simulink model "hw1b"  (R2022b)
settings: Solver=VariableStepAuto  StartTime=0.0  StopTime=200.0  FixedStep=0.1  MaxStep=0.1  MinStep=0.001  RelTol=1e-5  AbsTol=1e-8
undefined symbols (not defined in the file or in its folder): orbit, sat
settings Model: Creator=gagandeepthapar  LastModifiedBy=gagandeepthapar
settings SolverCC: InitialStep=0.1

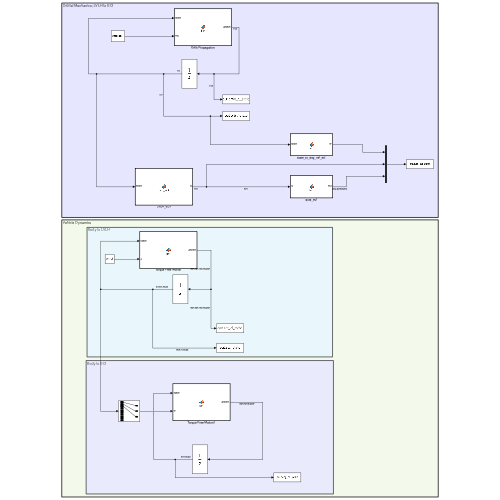
[thumbnail: Simulink's stored preview of the top-level diagram]
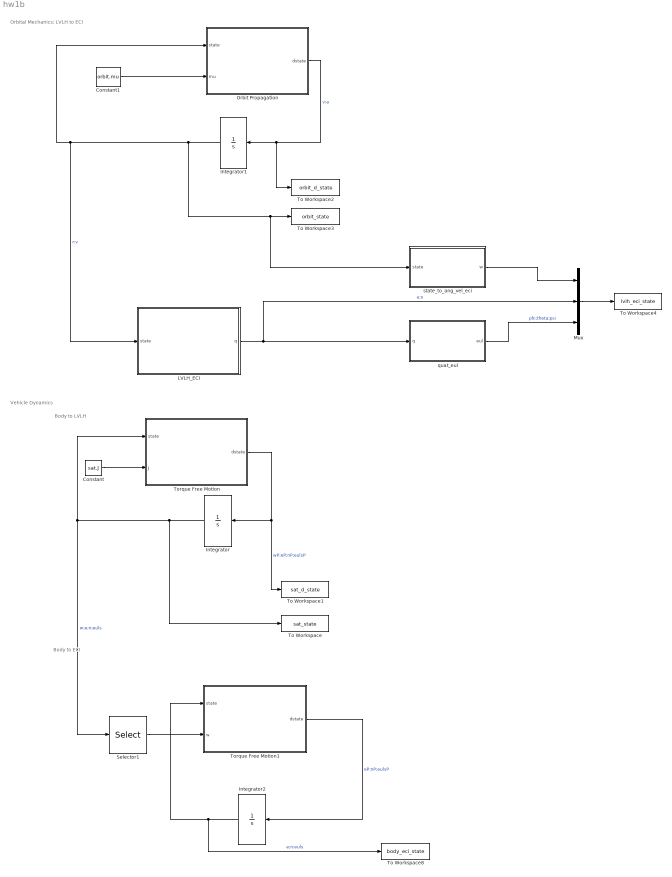
== system hw1b ==
  note: Body to LVLH
  note: Body to ECI
  note: Vehicle Dynamics
  note: Orbital Mechanics; LVLH to ECI
  Constant : Constant  Value=sat.J
  Constant1 : Constant  Value=orbit.mu
  Integrator : Integrator  InitialCondition=sat.state0
  Integrator1 : Integrator  InitialCondition=orbit.state0
  Integrator2 : Integrator  InitialCondition=sat.eci_state0
  LVLH_ECI : MATLAB Function  TreatAsAtomicUnit=on
  Mux : Mux  Inputs=3
  Orbit Propagation : MATLAB Function  TreatAsAtomicUnit=on
  Selector1 : Selector  InputPortWidth=10  IndexOptions=Index vector (dialog)  Indices=[1:3]  OutputSizes=1
  To Workspace : ToWorkspace  VariableName=sat_state  SampleTime=-1
      settings: Save2DSignal=2-D array (concatenate along first dimension)
  To Workspace1 : ToWorkspace  VariableName=sat_d_state  SampleTime=-1
      settings: Save2DSignal=2-D array (concatenate along first dimension)
  To Workspace2 : ToWorkspace  VariableName=orbit_d_state  SaveFormat=Timeseries  SampleTime=-1
  To Workspace3 : ToWorkspace  VariableName=orbit_state  SampleTime=-1
      settings: Save2DSignal=2-D array (concatenate along first dimension)
  To Workspace4 : ToWorkspace  VariableName=lvlh_eci_state  SampleTime=-1
      settings: Save2DSignal=2-D array (concatenate along first dimension)
  To Workspace8 : ToWorkspace  VariableName=body_eci_state  SampleTime=-1
      settings: Save2DSignal=2-D array (concatenate along first dimension)
  Torque Free Motion : MATLAB Function  TreatAsAtomicUnit=on
  Torque Free Motion1 : MATLAB Function  TreatAsAtomicUnit=on
  quat_eul : MATLAB Function  TreatAsAtomicUnit=on
  state_to_ang_vel_eci : MATLAB Function  TreatAsAtomicUnit=on
  wires:
  Constant/1 -> Torque Free Motion/2(J)
  Torque Free Motion/1(dstate) -> To Workspace1/1, Integrator/1  "wP;eP;nP;eulsP"
  Integrator/1 -> To Workspace/1, Torque Free Motion/1(state), Selector1/1  "w;e;n;euls"
  Constant1/1 -> Orbit Propagation/2(mu)
  Orbit Propagation/1(dstate) -> To Workspace2/1, Integrator1/1  "v;a"
  Integrator1/1 -> state_to_ang_vel_eci/1(state), To Workspace3/1, LVLH_ECI/1(state), Orbit Propagation/1(state)  "r;v"
  LVLH_ECI/1(q) -> Mux/2, quat_eul/1(q)  "e;n"
  quat_eul/1(eul) -> Mux/3  "phi;theta;psi"
  Torque Free Motion1/1(dstate) -> Integrator2/1  "eP;nP;eulsP"
  Integrator2/1 -> To Workspace8/1, Torque Free Motion1/1(state)  "e;n;euls"
  Selector1/1 -> Torque Free Motion1/2(w)
  state_to_ang_vel_eci/1(w) -> Mux/1
  Mux/1 -> To Workspace4/1

== matlab function hw1b/Torque Free Motion ==
  data: state input; dstate output; J input
function dstate = fcn(state, J)
    
    function wx = skewSymmetric(w)
        wx = [0, -1*w(3), w(2);
             w(3), 0, -1*w(1);
             -1*w(2), w(1), 0];
    end

    w = state(1:3);
    e = state(4:6);
    n = state(7);
    euls = state(8:10);

    wP = -1*J\(skewSymmetric(w)*J*w);
    eP = 0.5*(n*eye(3) + skewSymmetric(e))*w;
    nP = -0.5*e'*w;


    phi = euls(1);
    theta = euls(2);
    psi = euls(3);
    eulsP = 1/(cos(theta)) * [cos(theta), sin(phi)*sin(theta), cos(phi)*sin(theta);
                                0, cos(phi)*cos(theta), -1*sin(phi)*cos(theta);
                                0, sin(phi), cos(phi)] * w;


    dstate = [wP(1);wP(2);wP(3);eP(1);eP(2);eP(3);nP; eulsP(1); eulsP(2); eulsP(3)];


end

== matlab function hw1b/Orbit Propagation ==
  data: state input; dstate output; mu input
function dstate = fcn(state, mu)

    dstate = zeros(6,1);

    rx = state(1);
    ry = state(2);
    rz = state(3);
    vx = state(4);
    vy = state(5);
    vz = state(6);
    
    rad = norm([rx;ry;rz]);

    ax = -mu*rx/rad^3;
    ay = -mu*ry/rad^3;
    az = -mu*rz/rad^3;

    dstate(1:3) = [vx;vy;vz];
    dstate(4:6) = [ax;ay;az];

end

== matlab function hw1b/state_to_ang_vel_eci ==
  data: state input; w output
function w = fcn(state)

function Q = ECILVLH(R,V)

        if size(R) == [1 3]
            R = R';
        end
    
        if size(V) == [1 3]
            V = V';
        end
    
        z = -1*R / norm(R);
        y = -1 * cross(R,V) / norm(cross(R,V));
    
        x = cross(y,z);
    
        Q = [x,y,z]';

    end

r = [state(1);state(2);state(3)];
v = [state(4);state(5);state(6)];

w = ECILVLH(r,v) * cross(r,v)/(norm(r)^2);

w = [w(1);w(2);w(3)];

end

== matlab function hw1b/quat_eul ==
  data: q input; eul output
function eul = fcn(q)

    n = q(4);
    e = q(1:3);

    q = [n, e(1), e(2), e(3)];

    phi = atan2(2*(q(1)*q(2) + q(3)*q(4)), 1 - 2*(q(2)^2 + q(3)^2));
    theta = asin(2*(q(1)*q(3) - q(4)*q(2)));
    psi = atan2(2*(q(1)*q(4) + q(2)*q(3)), 1-2*(q(3)^2 + q(4)^2));

    eul = [phi; theta; psi];

end

== matlab function hw1b/Torque Free Motion1 ==
  data: state input; dstate output; w input
function dstate = fcn(state, w)
    
    function wx = skewSymmetric(w)
        wx = [0, -1*w(3), w(2);
             w(3), 0, -1*w(1);
             -1*w(2), w(1), 0];
    end

    e = state(1:3);
    n = state(4);
    euls = state(5:7);

    eP = 0.5*(n*eye(3) + skewSymmetric(e))*w;
    nP = -0.5*e'*w;


    phi = euls(1);
    theta = euls(2);
    psi = euls(3);
    eulsP = 1/(cos(theta)) * [cos(theta), sin(phi)*sin(theta), cos(phi)*sin(theta);
                                0, cos(phi)*cos(theta), -1*sin(phi)*cos(theta);
                                0, sin(phi), cos(phi)] * w;


    dstate = [eP(1);eP(2);eP(3);nP; eulsP(1); eulsP(2); eulsP(3)];


end

== matlab function hw1b/LVLH_ECI ==
  data: state input; q output
function q = lvlh_eci(state)

    function Q = ECILVLH(R,V)

    if size(R) == [1 3]
        R = R';
    end

    if size(V) == [1 3]
        V = V';
    end

    z = -1*R / norm(R);
    y = -1 * cross(R,V) / norm(cross(R,V));

    x = cross(y,z);

    Q = [x,y,z]';

    end

    function [e, n] = c2quat(C)
        e = zeros(3,1);
        n = 0.5 * sqrt(1 + trace(C));
        e(1) = 0.25 * (C(2,3) - C(3,2))/n;
        e(2) = 0.25 * (C(3,1) - C(1,3))/n;
        e(3) = 0.25 * (C(1,2) - C(2,1))/n;
    
    end

R = state(1:3);
V = state(4:6);

Q = ECILVLH(R,V);
[e,n] = c2quat(Q);

e = -1*e;
n = -1*n;

q = [e(1);e(2);e(3);n];

end
